simulink model "P1_DevDriv_z_krancowka_2015a_good_swingup"  (R2015a)
settings: Solver=ode5  SolverMode=SingleTasking  StartTime=0.0  StopTime=999  FixedStep=0.01  RelTol=1e-3  AbsTol=1e-6
undefined symbols (not defined in the file): Cntrl, g, J, K_reg, L, m, M, RTDAC4PCIBaseAddress
settings Model: SimulationMode=external  CovHtmlReporting=off  CovSFcnEnable=off  ExtModeTrigDuration=12000  ExtModeTrigDurationFloating=999000  ExtModeTrigLevel=0.400000  Creator=jims  LastModifiedBy=Student
settings DataIOCC: ExternalInput=[]  InitialState=[]  LimitDataPoints=off  MaxDataPoints=5000  SignalLoggingSaveFormat=ModelDataLogs  SaveOutput=off  SaveTime=off  SignalLoggingName=sigsOut
settings OptimizationCC: BooleanDataType=off  ExpressionDepthLimit=2147483647
settings DebuggingCC: SaveWithParameterizedLinksMsg=none  UnderspecifiedInitializationDetection=Classic  MergeDetectMultiDrivingBlocksExec=none  SignalResolutionControl=TryResolveAllWithWarning  MultiTaskDSMMsg=warning  MultiTaskCondExecSysMsg=none  IntegerOverflowMsg=none  FcnCallInpInsideContextMsg=EnableAllAsWarning  StateNameClashWarn=warning  IntegerSaturationMsg=none
settings HardwareCC: ProdBitPerLong=64  ProdBitPerPointer=64  ProdIntDivRoundTo=Zero  ProdEndianess=LittleEndian  ProdWordSize=64  ProdHWDeviceType=Intel->x86-64  TargetBitPerLong=64  TargetBitPerPointer=64  TargetIntDivRoundTo=Zero  TargetEndianess=LittleEndian  TargetWordSize=64  TargetHWDeviceType=Intel->x86-64
settings RTWCC: SystemTargetFile=rtwin.tlc  TemplateMakefile=rtwin.tmf  Description=Real-Time Windows Target  RTWCompilerOptimization=on
settings CodeAppCC: MaxIdLength=95
settings TargetCC: TargetPreCompLibLocation=C:\Program Files\MATLAB\R2015aSP1\toolbox\sldrt\lib\win64

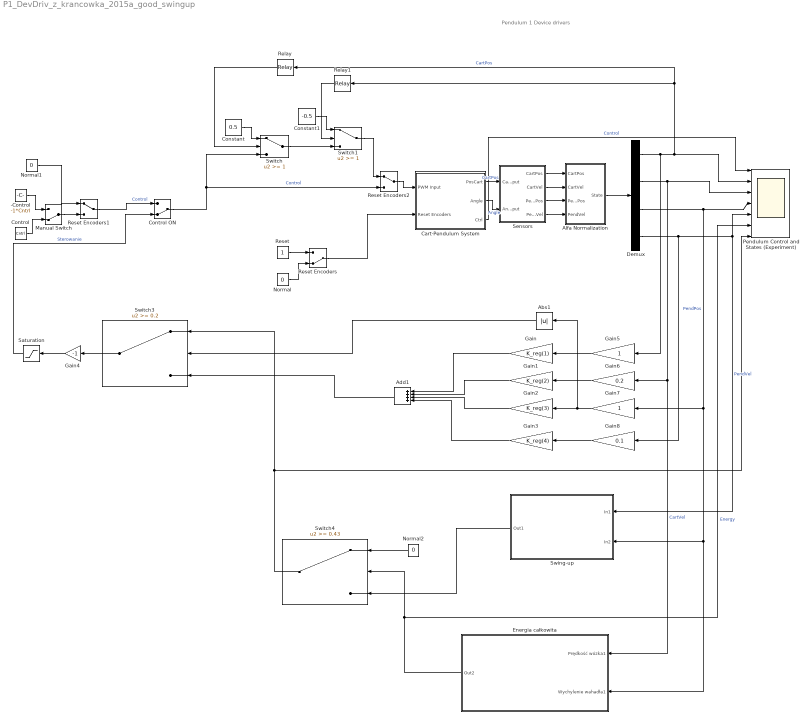
== system P1_DevDriv_z_krancowka_2015a_good_swingup ==
  note: Pendulum 1
      | Device drivers
  -Control : Constant  Value=-1*Cntrl
  Abs1 : Abs
  Add1 : Sum  Inputs=++++
  Alfa Normalization : Subsystem  mask(Choose mode:){pos=Inverted Pendulum}
      mask prompts: pos "Choose mode:"
      mask TypeOptions pos: Inverted Pendulum | Crane Controller
  Cart-Pendulum System : Subsystem  mask{BaseAddress=RTDAC4PCIBaseAddress(-1,-1), T0=0.01}
      mask prompts: BaseAddress "Base Address:"; T0 "Sampling Period:"
      mask Display: plot( [0.725 0.725], [1.05 0.375], 0.725+0.05*sin([0:0.5:7]), 0.325+0.05*cos([0:0.5:7]), [-0.3 -0.3], [-0.3 -0.3], [1.8 1.8], [1.8 1.8], [0.1 1.4], [0.95 0.95], [0.1 1.4], [0.92 0.92], [0.65 0.8], [1 1], [0.65 0.8], [1.1 1.1], [0.65 0.65], [1.1 1], [0.8 0.8], [1 1.1] )
  Constant : Constant  Value=0.5
  Constant1 : Constant  Value=-0.5
  Control : Constant  Value=Cntrl
  Control ON : ManualSwitch  CurrentSetting=0
  Demux : Demux
  Energia całkowita : Subsystem
  Gain : Gain  Gain=K_reg(1)
  Gain1 : Gain  Gain=K_reg(2)
  Gain2 : Gain  Gain=K_reg(3)
  Gain3 : Gain  Gain=K_reg(4)
  Gain4 : Gain  Gain=-1
  Gain5 : Gain
  Gain6 : Gain  Gain=0.2
  Gain7 : Gain
  Gain8 : Gain  Gain=0.1
  Manual Switch : ManualSwitch  CurrentSetting=0
  Normal : Constant  Value=0
  Normal1 : Constant  Value=0
  Normal2 : Constant  Value=0
  Pendulum Control and States (Experiment) : Scope  NumInputPorts=7
      settings: TimeRange=100  YMin=-0.5~-0.75~-5~-4~-25000~-1~-1  YMax=0.5~0.75~2~4~150000~10~1  SaveName=P1_ExpData  MaxDataPoints=50000
  Relay : Relay  OnSwitchValue=0.7  OffSwitchValue=0.6
  Relay1 : Relay  OnSwitchValue=-0.6  OffSwitchValue=-0.7  OnOutputValue=0  OffOutputValue=1
  Reset : Constant
  Reset Encoders : ManualSwitch  CurrentSetting=0
  Reset Encoders1 : ManualSwitch
  Reset Encoders2 : ManualSwitch
  Saturation : Saturate  UpperLimit=1  LowerLimit=-1
  Sensors : Subsystem  mask(PENDULUM Output){T0=0.01}
      mask prompts: T0 "Sample Time"
      mask help: PCL-812 PG Device Driver
  "Swing-up " : Subsystem
  Switch : Switch  Threshold=1
  Switch1 : Switch  Threshold=1
  Switch3 : Switch  Threshold=0.2
  Switch4 : Switch  Threshold=0.43
  wires:
  Reset Encoders/1 -> Cart-Pendulum System/2(Reset Encoders)
  Sensors/3(PendPos) -> Alfa Normalization/3(PendPos)
  Sensors/4(PendVel) -> Alfa Normalization/4(PendVel)
  Sensors/1(CartPos) -> Alfa Normalization/1(CartPos)
  Sensors/2(CartVel) -> Alfa Normalization/2(CartVel)
  Demux/1 -> Gain5/1, Pendulum Control and States (Experiment)/2, Relay/1, Relay1/1  "CartPos"
  Demux/2 -> Energia całkowita/1(Prędkość wózka1), Gain6/1, Pendulum Control and States (Experiment)/3  "CartVel"
  Demux/3 -> Energia całkowita/2(Wychylenie wahadła1), "Swing-up "/2(In2), Gain7/1, Pendulum Control and States (Experiment)/4  "PendPos"
  Demux/4 -> Gain8/1, "Swing-up "/1(In1), Pendulum Control and States (Experiment)/5  "PendVel"
  Cart-Pendulum System/1(PosCart) -> Sensors/1(CartPosInput)  "CartPos"
  Cart-Pendulum System/2(Angle) -> Sensors/2(AngleInput)  "Angle"
  Normal/1 -> Reset Encoders/2
  Reset/1 -> Reset Encoders/1
  Normal1/1 -> Reset Encoders1/1
  Manual Switch/1 -> Reset Encoders1/2
  Control/1 -> Manual Switch/2
  -Control/1 -> Manual Switch/1
  Control ON/1 -> Reset Encoders2/2, Switch/3  "Control"
  Relay/1 -> Switch/2
  Constant/1 -> Switch/1
  Reset Encoders2/1 -> Cart-Pendulum System/1(PWM Input)
  Relay1/1 -> Switch1/2
  Constant1/1 -> Switch1/1
  Switch/1 -> Switch1/3
  Switch1/1 -> Reset Encoders2/1
  Gain/1 -> Add1/1
  Gain1/1 -> Add1/2
  Gain2/1 -> Add1/3
  Gain3/1 -> Add1/4
  Gain4/1 -> Saturation/1
  Reset Encoders1/1 -> Control ON/1  "Control"
  Abs1/1 -> Switch3/2
  Alfa Normalization/1(State) -> Demux/1
  Cart-Pendulum System/3(Ctrl) -> Pendulum Control and States (Experiment)/1  "Control"
  Energia całkowita/1(Out2) -> Pendulum Control and States (Experiment)/6, Switch4/2  "Energy"
  Switch4/1 -> Pendulum Control and States (Experiment)/7, Switch3/1
  Switch3/1 -> Gain4/1
  Add1/1 -> Switch3/3
  Saturation/1 -> Control ON/2  "Sterowanie"
  "Swing-up "/1(Out1) -> Switch4/3
  Normal2/1 -> Switch4/1
  Gain5/1 -> Gain/1
  Gain6/1 -> Gain1/1
  Gain7/1 -> Abs1/1, Gain2/1
  Gain8/1 -> Gain3/1

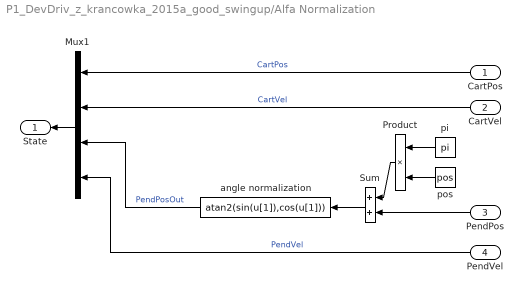
== system P1_DevDriv_z_krancowka_2015a_good_swingup/Alfa Normalization ==
  CartPos : Inport
  CartVel : Inport  Port=2
  PendPos : Inport  Port=3
  PendVel : Inport  Port=4
  Mux1 : Mux
  Product : Product  SaturateOnIntegerOverflow=on  InputSameDT=on  OutDataTypeStr=Inherit: Same as first input
  Sum : Sum  SaturateOnIntegerOverflow=on  InputSameDT=on  OutDataTypeStr=Inherit: Same as first input
  angle normalization : Fcn  Expr=atan2(sin(u[1]),cos(u[1]))
  pi : Constant  Value=pi
  pos : Constant  Value=pos
  State : Outport  InitialOutput=0
  wires:
  angle normalization/1 -> Mux1/3  "PendPosOut"
  PendVel/1 -> Mux1/4  "PendVel"
  CartVel/1 -> Mux1/2  "CartVel"
  CartPos/1 -> Mux1/1  "CartPos"
  Mux1/1 -> State/1
  Sum/1 -> angle normalization/1
  PendPos/1 -> Sum/2
  pi/1 -> Product/1
  pos/1 -> Product/2
  Product/1 -> Sum/1

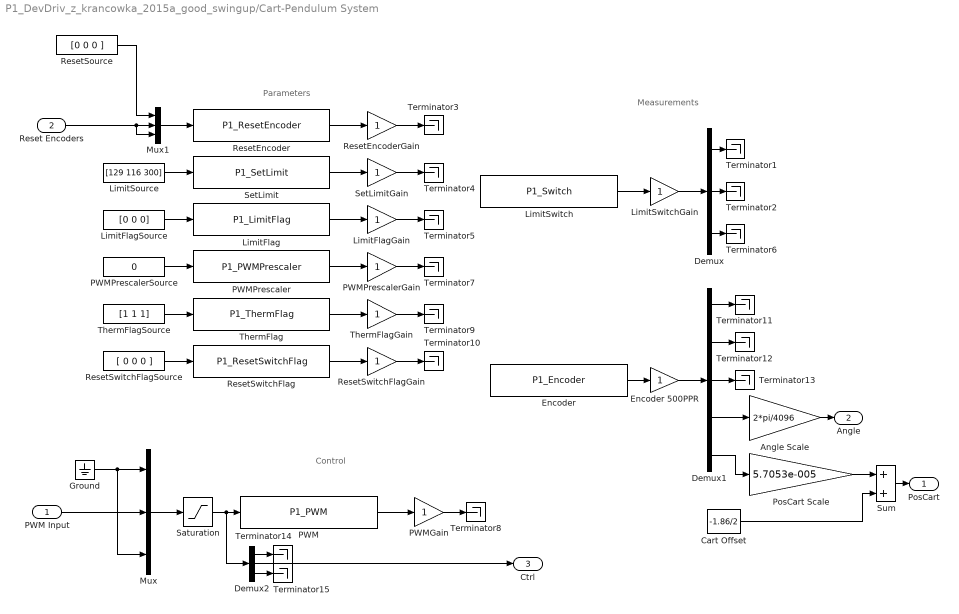
== system P1_DevDriv_z_krancowka_2015a_good_swingup/Cart-Pendulum System ==
  note: Measurements
  note: Control
  note: Parameters
  PWM Input : Inport
  Reset Encoders : Inport  Port=2
  Angle Scale : Gain  Gain=2*pi/4096  OutDataTypeStr=Inherit: Same as input  ParamDataTypeStr=Inherit: Same as input
  Cart Offset : Constant  Value=-1.86/2
  Demux : Demux  Outputs=3
  Demux1 : Demux  Outputs=5
  Demux2 : Demux  Outputs=3
  Encoder : S-Function  FunctionName=P1_Encoder  Parameters=BaseAddress, T0
  Encoder 500PPR : Gain  SaturateOnIntegerOverflow=on  OutDataTypeStr=Inherit: Same as input  ParamDataTypeStr=Inherit: Same as input
  Ground : Ground
  LimitFlag : S-Function  FunctionName=P1_LimitFlag  Parameters=BaseAddress, T0
  LimitFlagGain : Gain  SaturateOnIntegerOverflow=on  OutDataTypeStr=Inherit: Same as input  ParamDataTypeStr=Inherit: Same as input
  LimitFlagSource : Constant  Value=[0 0 0]
  LimitSource : Constant  Value=[129 116 300]
  LimitSwitch : S-Function  FunctionName=P1_Switch  Parameters=BaseAddress, T0
  LimitSwitchGain : Gain  SaturateOnIntegerOverflow=on  OutDataTypeStr=Inherit: Same as input  ParamDataTypeStr=Inherit: Same as input
  Mux : Mux  Inputs=3
  Mux1 : Mux  Inputs=[3 1 1]
  PWM : S-Function  FunctionName=P1_PWM  Parameters=BaseAddress, T0
  PWMGain : Gain  SaturateOnIntegerOverflow=on  OutDataTypeStr=Inherit: Same as input  ParamDataTypeStr=Inherit: Same as input
  PWMPrescaler : S-Function  FunctionName=P1_PWMPrescaler  Parameters=BaseAddress, T0
  PWMPrescalerGain : Gain  SaturateOnIntegerOverflow=on  OutDataTypeStr=Inherit: Same as input  ParamDataTypeStr=Inherit: Same as input
  PWMPrescalerSource : Constant  Value=0
  PosCart Scale : Gain  Gain=5.7053e-005  OutDataTypeStr=Inherit: Same as input  ParamDataTypeStr=Inherit: Same as input
  ResetEncoder : S-Function  FunctionName=P1_ResetEncoder  Parameters=BaseAddress, T0
  ResetEncoderGain : Gain  SaturateOnIntegerOverflow=on  OutDataTypeStr=Inherit: Same as input  ParamDataTypeStr=Inherit: Same as input
  ResetSource : Constant  Value=[0 0 0 ]
  "ResetSwitchFlag " : S-Function  FunctionName=P1_ResetSwitchFlag  Parameters=BaseAddress, T0
  ResetSwitchFlagGain : Gain  SaturateOnIntegerOverflow=on  OutDataTypeStr=Inherit: Same as input  ParamDataTypeStr=Inherit: Same as input
  ResetSwitchFlagSource : Constant  Value=[ 0 0 0 ]
  Saturation : Saturate
  SetLimit : S-Function  FunctionName=P1_SetLimit  Parameters=BaseAddress, T0
  SetLimitGain : Gain  SaturateOnIntegerOverflow=on  OutDataTypeStr=Inherit: Same as input  ParamDataTypeStr=Inherit: Same as input
  Sum : Sum  SaturateOnIntegerOverflow=on  InputSameDT=on  OutDataTypeStr=Inherit: Same as first input
  Terminator{1..15} (15 alike) : Terminator
  "ThermFlag " : S-Function  FunctionName=P1_ThermFlag  Parameters=BaseAddress, T0
  ThermFlagGain : Gain  SaturateOnIntegerOverflow=on  OutDataTypeStr=Inherit: Same as input  ParamDataTypeStr=Inherit: Same as input
  ThermFlagSource : Constant  Value=[1 1 1]
  PosCart : Outport  InitialOutput=0
  Angle : Outport  Port=2  InitialOutput=0
  Ctrl : Outport  Port=3  InitialOutput=0
  wires:
  Demux1/1 -> Terminator11/1
  Demux1/2 -> Terminator12/1
  Demux1/3 -> Terminator13/1
  Demux1/4 -> Angle Scale/1
  Demux1/5 -> PosCart Scale/1
  Angle Scale/1 -> Angle/1
  Demux/3 -> Terminator6/1
  Demux/2 -> Terminator2/1
  Demux/1 -> Terminator1/1
  LimitSwitchGain/1 -> Demux/1
  LimitSwitch/1 -> LimitSwitchGain/1
  Ground/1 -> Mux/1, Mux/3
  PWM Input/1 -> Mux/2
  ResetSwitchFlagGain/1 -> Terminator10/1
  ThermFlagGain/1 -> Terminator9/1
  PWMPrescalerGain/1 -> Terminator7/1
  LimitFlagGain/1 -> Terminator5/1
  SetLimitGain/1 -> Terminator4/1
  ResetEncoderGain/1 -> Terminator3/1
  ResetSwitchFlagSource/1 -> "ResetSwitchFlag "/1
  ThermFlagSource/1 -> "ThermFlag "/1
  PWMPrescalerSource/1 -> PWMPrescaler/1
  LimitFlagSource/1 -> LimitFlag/1
  LimitSource/1 -> SetLimit/1
  "ResetSwitchFlag "/1 -> ResetSwitchFlagGain/1
  "ThermFlag "/1 -> ThermFlagGain/1
  PWMPrescaler/1 -> PWMPrescalerGain/1
  LimitFlag/1 -> LimitFlagGain/1
  SetLimit/1 -> SetLimitGain/1
  ResetEncoder/1 -> ResetEncoderGain/1
  PWM/1 -> PWMGain/1
  Mux/1 -> Saturation/1
  Saturation/1 -> Demux2/1, PWM/1
  Encoder/1 -> Encoder 500PPR/1
  Encoder 500PPR/1 -> Demux1/1
  Mux1/1 -> ResetEncoder/1
  ResetSource/1 -> Mux1/1
  Reset Encoders/1 -> Mux1/2, Mux1/3
  PosCart Scale/1 -> Sum/1
  Sum/1 -> PosCart/1
  Cart Offset/1 -> Sum/2
  PWMGain/1 -> Terminator8/1
  Demux2/2 -> Ctrl/1
  Demux2/1 -> Terminator14/1
  Demux2/3 -> Terminator15/1

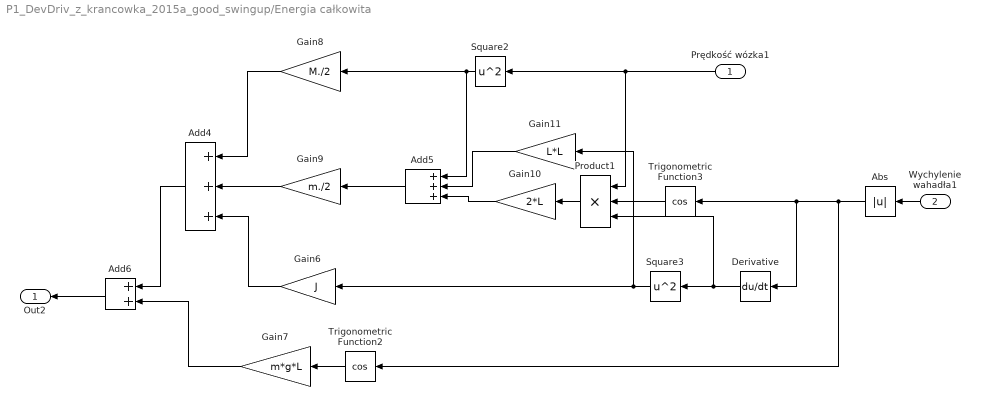
== system P1_DevDriv_z_krancowka_2015a_good_swingup/Energia całkowita ==
  Prędkość wózka1 : Inport
  Wychylenie wahadła1 : Inport  Port=2
  Abs : Abs
  Add4 : Sum  Inputs=+++
  Add5 : Sum  Inputs=+++
  Add6 : Sum
  Derivative : Derivative
  Gain10 : Gain  Gain=2*L
  Gain11 : Gain  Gain=L*L
  Gain6 : Gain  Gain=J
  Gain7 : Gain  Gain=m*g*L
  Gain8 : Gain  Gain=M./2
  Gain9 : Gain  Gain=m./2
  Product1 : Product  Inputs=3
  Square2 : Math  Operator=square  SaturateOnIntegerOverflow=on
  Square3 : Math  Operator=square  SaturateOnIntegerOverflow=on
  Trigonometric Function2 : Trigonometry  Operator=cos
  Trigonometric Function3 : Trigonometry  Operator=cos
  Out2 : Outport
  wires:
  Trigonometric Function2/1 -> Gain7/1
  Gain7/1 -> Add6/2
  Gain6/1 -> Add4/3
  Add6/1 -> Out2/1
  Wychylenie wahadła1/1 -> Abs/1
  Gain8/1 -> Add4/1
  Square2/1 -> Add5/1, Gain8/1
  Gain9/1 -> Add4/2
  Add5/1 -> Gain9/1
  Gain10/1 -> Add5/3
  Gain11/1 -> Add5/2
  Product1/1 -> Gain10/1
  Trigonometric Function3/1 -> Product1/2
  Prędkość wózka1/1 -> Square2/1, Product1/1
  Add4/1 -> Add6/1
  Derivative/1 -> Product1/3, Square3/1
  Square3/1 -> Gain11/1, Gain6/1
  Abs/1 -> Trigonometric Function2/1, Derivative/1, Trigonometric Function3/1

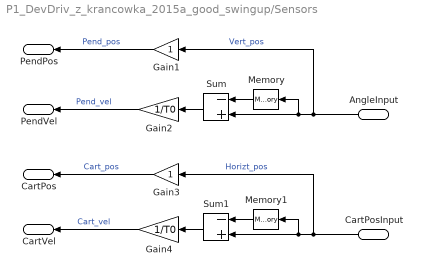
== system P1_DevDriv_z_krancowka_2015a_good_swingup/Sensors ==
  CartPosInput : Inport
  AngleInput : Inport  Port=2
  Gain1 : Gain  SaturateOnIntegerOverflow=on  OutDataTypeStr=Inherit: Same as input  ParamDataTypeStr=Inherit: Same as input
  Gain2 : Gain  Gain=1/T0  SaturateOnIntegerOverflow=on  OutDataTypeStr=Inherit: Same as input  ParamDataTypeStr=Inherit: Same as input
  Gain3 : Gain  SaturateOnIntegerOverflow=on  OutDataTypeStr=Inherit: Same as input  ParamDataTypeStr=Inherit: Same as input
  Gain4 : Gain  Gain=1/T0  SaturateOnIntegerOverflow=on  OutDataTypeStr=Inherit: Same as input  ParamDataTypeStr=Inherit: Same as input
  Memory : Memory
  Memory1 : Memory
  Sum : Sum  Inputs=-+  SaturateOnIntegerOverflow=on  InputSameDT=on  OutDataTypeStr=Inherit: Same as first input
  Sum1 : Sum  Inputs=-+  SaturateOnIntegerOverflow=on  InputSameDT=on  OutDataTypeStr=Inherit: Same as first input
  CartPos : Outport  InitialOutput=0
  CartVel : Outport  Port=2  InitialOutput=0
  PendPos : Outport  Port=3  InitialOutput=0
  PendVel : Outport  Port=4  InitialOutput=0
  wires:
  Gain4/1 -> CartVel/1  "Cart_vel"
  Sum1/1 -> Gain4/1
  Memory1/1 -> Sum1/1
  Sum/1 -> Gain2/1
  Memory/1 -> Sum/1
  CartPosInput/1 -> Memory1/1, Sum1/2, Gain3/1  "Horizt_pos"
  AngleInput/1 -> Memory/1, Sum/2, Gain1/1  "Vert_pos"
  Gain2/1 -> PendVel/1  "Pend_vel"
  Gain1/1 -> PendPos/1  "Pend_pos"
  Gain3/1 -> CartPos/1  "Cart_pos"

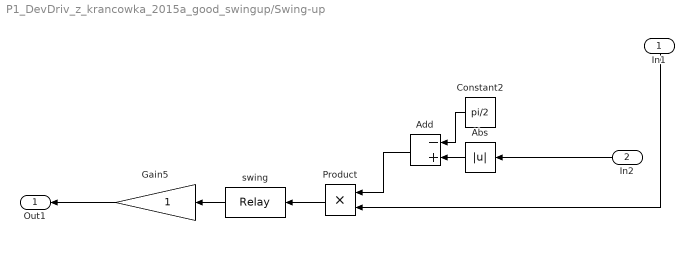
== system P1_DevDriv_z_krancowka_2015a_good_swingup/Swing-up  ==
  In1 : Inport
  In2 : Inport  Port=2
  Abs : Abs
  Add : Sum  Inputs=-+
  Constant2 : Constant  Value=pi/2
  Gain5 : Gain
  Product : Product
  swing : Relay  OffOutputValue=-1
  Out1 : Outport
  wires:
  In1/1 -> Product/2
  In2/1 -> Abs/1
  Product/1 -> swing/1
  swing/1 -> Gain5/1
  Gain5/1 -> Out1/1
  Constant2/1 -> Add/1
  Abs/1 -> Add/2
  Add/1 -> Product/1
